simulink model "ctrl_student_HI_backup"  (R2015a)
settings: Solver=ode4  StartTime=0.0  StopTime=inf  FixedStep=0.01  RelTol=1e-3
undefined symbols (not defined in the file or in its folder): now, Par
(part 2 of 2)

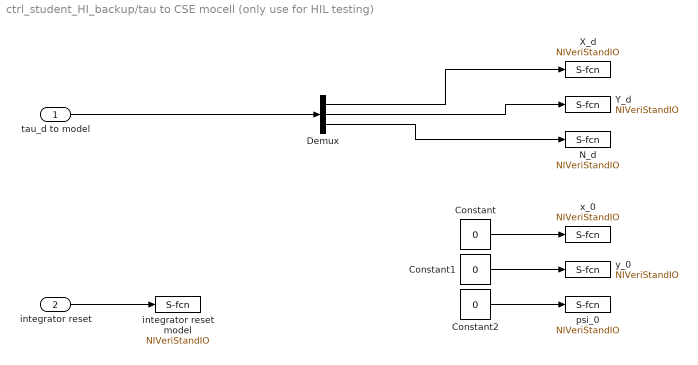
== system ctrl_student_HI_backup/tau to CSE mocell (only use for HIL testing) ==
  tau_d to model : Inport
  integrator reset : Inport  Port=2
  Constant : Constant  Value=0
  Constant1 : Constant  Value=0
  Constant2 : Constant  Value=0
  Demux : Demux  Outputs=3
  N_d : S-Function  Priority=2  FunctionName=NIVeriStandIO  Parameters=width dtype portnum stime stype btype  mask(NI VeriStand Outport){portnum=2, width=-1, stime=-1, dtype=auto, stype=auto, btype=0}
      mask prompts: portnum "Port number:"; width "Port dimensions (-1 for dynamically sized):"; stime "Sample time (-1 for inherited):"; dtype "Data type:"; stype "Signal type:"; btype "Block type:"
      mask help: Use this outport on any level of nested subsystems to allow NI VeriStand software to map signals to it.
      mask init:
      | NIVeriStandIO_init;
      settings: CopyFcn=NIVeriStand_MDL_functions('', 'IO_copy');  DeleteFcn=NIVeriStand_MDL_functions('', 'IO_delete');  MoveFcn=set_param(gcb, 'Mask', 'on');
      mask Callback portnum: NIVeriStand_MDL_functions('', 'IO_setportnum');
      mask TypeOptions dtype: auto | double | single | int8 | uint8 | int16 | uint16 | int32 | uint32 | boolean
      mask Callback dtype: NIVeriStand_MDL_functions('', 'IO_booleansignal');
      mask TypeOptions stype: auto | real | complex
      mask Display:
      | patch([-x x], [-y y], [.90980 .81960 .32156]);
      | plot([xrad -x x xrad], [yrad -y y yrad]);
      | fprintf('NI Out%d', portnum);
  X_d : S-Function  Priority=1  FunctionName=NIVeriStandIO  Parameters=width dtype portnum stime stype btype  mask(NI VeriStand Outport){portnum=1, width=-1, stime=-1, dtype=auto, stype=auto, btype=0}
      mask prompts: portnum "Port number:"; width "Port dimensions (-1 for dynamically sized):"; stime "Sample time (-1 for inherited):"; dtype "Data type:"; stype "Signal type:"; btype "Block type:"
      mask help: Use this outport on any level of nested subsystems to allow NI VeriStand software to map signals to it.
      mask init:
      | NIVeriStandIO_init;
      settings: CopyFcn=NIVeriStand_MDL_functions('', 'IO_copy');  DeleteFcn=NIVeriStand_MDL_functions('', 'IO_delete');  MoveFcn=set_param(gcb, 'Mask', 'on');
      mask Callback portnum: NIVeriStand_MDL_functions('', 'IO_setportnum');
      mask TypeOptions dtype: auto | double | single | int8 | uint8 | int16 | uint16 | int32 | uint32 | boolean
      mask Callback dtype: NIVeriStand_MDL_functions('', 'IO_booleansignal');
      mask TypeOptions stype: auto | real | complex
      mask Display:
      | patch([-x x], [-y y], [.90980 .81960 .32156]);
      | plot([xrad -x x xrad], [yrad -y y yrad]);
      | fprintf('NI Out%d', portnum);
  Y_d : S-Function  Priority=3  FunctionName=NIVeriStandIO  Parameters=width dtype portnum stime stype btype  mask(NI VeriStand Outport){portnum=3, width=-1, stime=-1, dtype=auto, stype=auto, btype=0}
      mask prompts: portnum "Port number:"; width "Port dimensions (-1 for dynamically sized):"; stime "Sample time (-1 for inherited):"; dtype "Data type:"; stype "Signal type:"; btype "Block type:"
      mask help: Use this outport on any level of nested subsystems to allow NI VeriStand software to map signals to it.
      mask init:
      | NIVeriStandIO_init;
      settings: CopyFcn=NIVeriStand_MDL_functions('', 'IO_copy');  DeleteFcn=NIVeriStand_MDL_functions('', 'IO_delete');  MoveFcn=set_param(gcb, 'Mask', 'on');
      mask Callback portnum: NIVeriStand_MDL_functions('', 'IO_setportnum');
      mask TypeOptions dtype: auto | double | single | int8 | uint8 | int16 | uint16 | int32 | uint32 | boolean
      mask Callback dtype: NIVeriStand_MDL_functions('', 'IO_booleansignal');
      mask TypeOptions stype: auto | real | complex
      mask Display:
      | patch([-x x], [-y y], [.90980 .81960 .32156]);
      | plot([xrad -x x xrad], [yrad -y y yrad]);
      | fprintf('NI Out%d', portnum);
  integrator reset model : S-Function  Priority=7  FunctionName=NIVeriStandIO  Parameters=width dtype portnum stime stype btype  mask(NI VeriStand Outport){portnum=7, width=-1, stime=-1, dtype=auto, stype=auto, btype=0}
      mask prompts: portnum "Port number:"; width "Port dimensions (-1 for dynamically sized):"; stime "Sample time (-1 for inherited):"; dtype "Data type:"; stype "Signal type:"; btype "Block type:"
      mask help: Use this outport on any level of nested subsystems to allow NI VeriStand software to map signals to it.
      mask init:
      | NIVeriStandIO_init;
      settings: CopyFcn=NIVeriStand_MDL_functions('', 'IO_copy');  DeleteFcn=NIVeriStand_MDL_functions('', 'IO_delete');  MoveFcn=set_param(gcb, 'Mask', 'on');
      mask Callback portnum: NIVeriStand_MDL_functions('', 'IO_setportnum');
      mask TypeOptions dtype: auto | double | single | int8 | uint8 | int16 | uint16 | int32 | uint32 | boolean
      mask Callback dtype: NIVeriStand_MDL_functions('', 'IO_booleansignal');
      mask TypeOptions stype: auto | real | complex
      mask Display:
      | patch([-x x], [-y y], [.90980 .81960 .32156]);
      | plot([xrad -x x xrad], [yrad -y y yrad]);
      | fprintf('NI Out%d', portnum);
  "psi_0 " : S-Function  Priority=4  FunctionName=NIVeriStandIO  Parameters=width dtype portnum stime stype btype  mask(NI VeriStand Outport){portnum=4, width=-1, stime=-1, dtype=auto, stype=auto, btype=0}
      mask prompts: portnum "Port number:"; width "Port dimensions (-1 for dynamically sized):"; stime "Sample time (-1 for inherited):"; dtype "Data type:"; stype "Signal type:"; btype "Block type:"
      mask help: Use this outport on any level of nested subsystems to allow NI VeriStand software to map signals to it.
      mask init:
      | NIVeriStandIO_init;
      settings: CopyFcn=NIVeriStand_MDL_functions('', 'IO_copy');  DeleteFcn=NIVeriStand_MDL_functions('', 'IO_delete');  MoveFcn=set_param(gcb, 'Mask', 'on');
      mask Callback portnum: NIVeriStand_MDL_functions('', 'IO_setportnum');
      mask TypeOptions dtype: auto | double | single | int8 | uint8 | int16 | uint16 | int32 | uint32 | boolean
      mask Callback dtype: NIVeriStand_MDL_functions('', 'IO_booleansignal');
      mask TypeOptions stype: auto | real | complex
      mask Display:
      | patch([-x x], [-y y], [.90980 .81960 .32156]);
      | plot([xrad -x x xrad], [yrad -y y yrad]);
      | fprintf('NI Out%d', portnum);
  x_0 : S-Function  Priority=5  FunctionName=NIVeriStandIO  Parameters=width dtype portnum stime stype btype  mask(NI VeriStand Outport){portnum=5, width=-1, stime=-1, dtype=auto, stype=auto, btype=0}
      mask prompts: portnum "Port number:"; width "Port dimensions (-1 for dynamically sized):"; stime "Sample time (-1 for inherited):"; dtype "Data type:"; stype "Signal type:"; btype "Block type:"
      mask help: Use this outport on any level of nested subsystems to allow NI VeriStand software to map signals to it.
      mask init:
      | NIVeriStandIO_init;
      settings: CopyFcn=NIVeriStand_MDL_functions('', 'IO_copy');  DeleteFcn=NIVeriStand_MDL_functions('', 'IO_delete');  MoveFcn=set_param(gcb, 'Mask', 'on');
      mask Callback portnum: NIVeriStand_MDL_functions('', 'IO_setportnum');
      mask TypeOptions dtype: auto | double | single | int8 | uint8 | int16 | uint16 | int32 | uint32 | boolean
      mask Callback dtype: NIVeriStand_MDL_functions('', 'IO_booleansignal');
      mask TypeOptions stype: auto | real | complex
      mask Display:
      | patch([-x x], [-y y], [.90980 .81960 .32156]);
      | plot([xrad -x x xrad], [yrad -y y yrad]);
      | fprintf('NI Out%d', portnum);
  y_0 : S-Function  Priority=6  FunctionName=NIVeriStandIO  Parameters=width dtype portnum stime stype btype  mask(NI VeriStand Outport){portnum=6, width=-1, stime=-1, dtype=auto, stype=auto, btype=0}
      mask prompts: portnum "Port number:"; width "Port dimensions (-1 for dynamically sized):"; stime "Sample time (-1 for inherited):"; dtype "Data type:"; stype "Signal type:"; btype "Block type:"
      mask help: Use this outport on any level of nested subsystems to allow NI VeriStand software to map signals to it.
      mask init:
      | NIVeriStandIO_init;
      settings: CopyFcn=NIVeriStand_MDL_functions('', 'IO_copy');  DeleteFcn=NIVeriStand_MDL_functions('', 'IO_delete');  MoveFcn=set_param(gcb, 'Mask', 'on');
      mask Callback portnum: NIVeriStand_MDL_functions('', 'IO_setportnum');
      mask TypeOptions dtype: auto | double | single | int8 | uint8 | int16 | uint16 | int32 | uint32 | boolean
      mask Callback dtype: NIVeriStand_MDL_functions('', 'IO_booleansignal');
      mask TypeOptions stype: auto | real | complex
      mask Display:
      | patch([-x x], [-y y], [.90980 .81960 .32156]);
      | plot([xrad -x x xrad], [yrad -y y yrad]);
      | fprintf('NI Out%d', portnum);
  wires:
  tau_d to model/1 -> Demux/1
  Demux/1 -> X_d/1
  Demux/2 -> Y_d/1
  Demux/3 -> N_d/1
  Constant2/1 -> "psi_0 "/1
  Constant1/1 -> y_0/1
  Constant/1 -> x_0/1
  integrator reset/1 -> integrator reset model/1

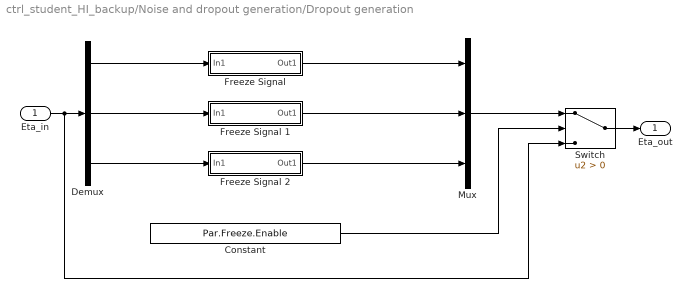
== system ctrl_student_HI_backup/Noise and dropout generation/Dropout generation ==
  Eta_in : Inport
  Constant : Constant  Value=Par.Freeze.Enable
  Demux : Demux  Outputs=3
  "Freeze Signal " : Subsystem
  Freeze Signal 1 : Subsystem
  Freeze Signal 2 : Subsystem
  Mux : Mux  Inputs=3
  Switch : Switch  Criteria=u2 > Threshold
  Eta_out : Outport
  wires:
  Eta_in/1 -> Switch/3, Demux/1
  Mux/1 -> Switch/1
  Demux/1 -> "Freeze Signal "/1(In1)
  "Freeze Signal "/1(Out1) -> Mux/1
  Freeze Signal 1/1(Out1) -> Mux/2
  Demux/2 -> Freeze Signal 1/1(In1)
  Demux/3 -> Freeze Signal 2/1(In1)
  Freeze Signal 2/1(Out1) -> Mux/3
  Constant/1 -> Switch/2
  Switch/1 -> Eta_out/1

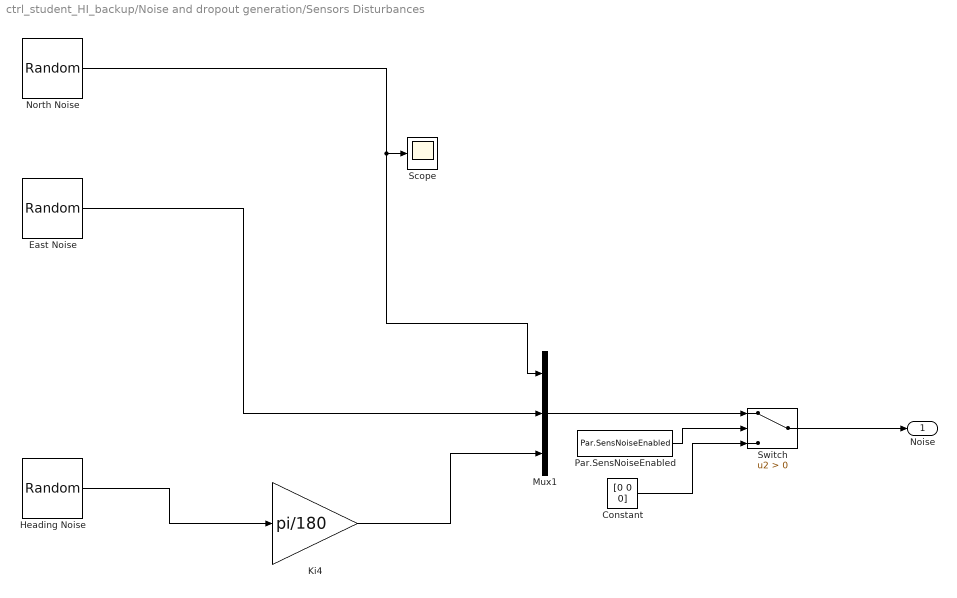
== system ctrl_student_HI_backup/Noise and dropout generation/Sensors Disturbances ==
  Constant : Constant  Value=[0 0 0]
  East Noise : RandomNumber  DisableCoverage=on  Variance=Par.Noise.Power  Seed=ceil(abs(5*round(abs(now*1e6 - fix(now*1e6))*1e5)))  SampleTime=Par.Sample_time  VectorParams1D=off
  Heading Noise : RandomNumber  DisableCoverage=on  Variance=Par.Noise.Power  Seed=ceil(abs(11*round(abs(now*1e6 - fix(now*1e6))*1e5)))  SampleTime=Par.Sample_time
  Ki4 : Gain  Gain=pi/180  RndMeth=Nearest
  Mux1 : Mux  Inputs=3
  North Noise : RandomNumber  DisableCoverage=on  Variance=Par.Noise.Power  Seed=ceil(abs(3*round(abs(now*1e6 - fix(now*1e6))*1e5)))  SampleTime=Par.Sample_time
  Par.SensNoiseEnabled : Constant  Value=Par.SensNoiseEnabled
  Scope : Scope
      settings: YMin=-0.51365  YMax=0.47143  SaveName=ScopeData2
  Switch : Switch  Criteria=u2 > Threshold
  Noise : Outport
  wires:
  East Noise/1 -> Mux1/2
  North Noise/1 -> Mux1/1, Scope/1
  Par.SensNoiseEnabled/1 -> Switch/2
  Switch/1 -> Noise/1
  Constant/1 -> Switch/3
  Mux1/1 -> Switch/1
  Heading Noise/1 -> Ki4/1
  Ki4/1 -> Mux1/3

== system ctrl_student_HI_backup/Signal Dropout detection/r ==
  detect droput : Inport
  nu : Inport  Port=2
  eta : Inport  Port=3
  Integrator : Integrator  ExternalReset=rising  InitialConditionSource=external
  Switch : Switch  Criteria=u2 ~= 0
  new_eta : Outport
  wires:
  Switch/1 -> new_eta/1
  nu/1 -> Integrator/1
  eta/1 -> Switch/3, Integrator/3
  detect droput/1 -> Switch/2, Integrator/2
  Integrator/1 -> Switch/1

== system ctrl_student_HI_backup/Signal Dropout detection/x ==
  detect droput : Inport
  nu : Inport  Port=2
  eta : Inport  Port=3
  Integrator : Integrator  ExternalReset=rising  InitialConditionSource=external
  Switch : Switch  Criteria=u2 ~= 0
  new_eta : Outport
  wires:
  Switch/1 -> new_eta/1
  nu/1 -> Integrator/1
  eta/1 -> Switch/3, Integrator/3
  detect droput/1 -> Switch/2, Integrator/2
  Integrator/1 -> Switch/1

== system ctrl_student_HI_backup/Signal Dropout detection/y ==
  detect droput : Inport
  nu : Inport  Port=2
  eta : Inport  Port=3
  Integrator : Integrator  ExternalReset=rising  InitialConditionSource=external
  Switch : Switch  Criteria=u2 ~= 0
  new_eta : Outport
  wires:
  Switch/1 -> new_eta/1
  nu/1 -> Integrator/1
  eta/1 -> Switch/3, Integrator/3
  detect droput/1 -> Switch/2, Integrator/2
  Integrator/1 -> Switch/1

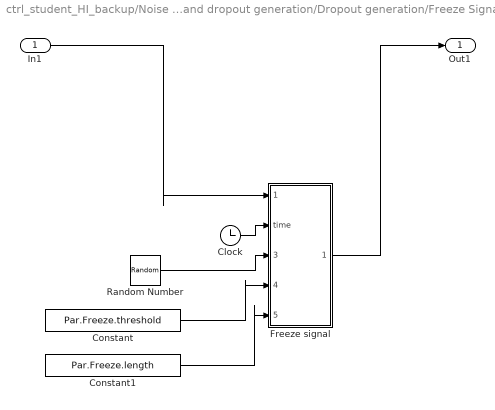
== system ctrl_student_HI_backup/Noise and dropout generation/Dropout generation/Freeze Signal  ==
  In1 : Inport
  Clock : Clock
  Constant : Constant  Value=Par.Freeze.threshold
  Constant1 : Constant  Value=Par.Freeze.length
  Freeze signal : MATLAB Function  TreatAsAtomicUnit=on
  Random Number : RandomNumber  Seed=ceil(abs(5*round(abs(now*1e6 - fix(now*1e6))*1e5)))  SampleTime=Par.Sample_time
  Out1 : Outport
  wires:
  Constant1/1 -> Freeze signal/5(length)
  In1/1 -> Freeze signal/1(eta_in)
  Freeze signal/1(eta_out) -> Out1/1
  Constant/1 -> Freeze signal/4(threshold)
  Clock/1 -> Freeze signal/2(time)
  Random Number/1 -> Freeze signal/3(random_value)

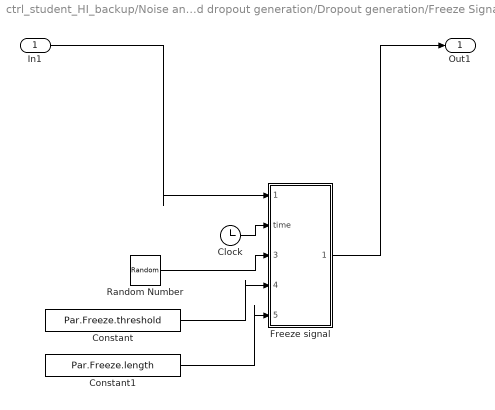
== system ctrl_student_HI_backup/Noise and dropout generation/Dropout generation/Freeze Signal 1 ==
  In1 : Inport
  Clock : Clock
  Constant : Constant  Value=Par.Freeze.threshold
  Constant1 : Constant  Value=Par.Freeze.length
  Freeze signal : MATLAB Function  TreatAsAtomicUnit=on
  Random Number : RandomNumber  Seed=ceil(abs(5*round(abs(now*1e6 - fix(now*1e6))*1e5)))  SampleTime=Par.Sample_time
  Out1 : Outport
  wires:
  Constant1/1 -> Freeze signal/5(length)
  In1/1 -> Freeze signal/1(eta_in)
  Freeze signal/1(eta_out) -> Out1/1
  Constant/1 -> Freeze signal/4(threshold)
  Clock/1 -> Freeze signal/2(time)
  Random Number/1 -> Freeze signal/3(random_value)

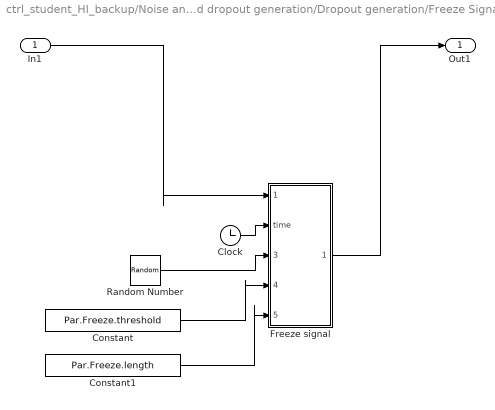
== system ctrl_student_HI_backup/Noise and dropout generation/Dropout generation/Freeze Signal 2 ==
  In1 : Inport
  Clock : Clock
  Constant : Constant  Value=Par.Freeze.threshold
  Constant1 : Constant  Value=Par.Freeze.length
  Freeze signal : MATLAB Function  TreatAsAtomicUnit=on
  Random Number : RandomNumber  Seed=ceil(abs(5*round(abs(now*1e6 - fix(now*1e6))*1e5)))  SampleTime=Par.Sample_time
  Out1 : Outport
  wires:
  Constant1/1 -> Freeze signal/5(length)
  In1/1 -> Freeze signal/1(eta_in)
  Freeze signal/1(eta_out) -> Out1/1
  Constant/1 -> Freeze signal/4(threshold)
  Clock/1 -> Freeze signal/2(time)
  Random Number/1 -> Freeze signal/3(random_value)

== matlab function ctrl_student_HI_backup/Thrust Allocation/MATLAB Function ==
  data: X input; u output; Y input; N input; invT input
function u = fcn(X, Y, N, invT)
%#codegen
u = [0 0 0]';
u = invT*[X, Y, N]';

== matlab function ctrl_student_HI_backup/Surge Observer/inside of integral ==
  data: psi input; k_psi input; X input; u_hat input; integral output
function integral = fcn(psi, k_psi, X, u_hat)
%#codegen
X_u = -.6555;
X_uu = .3545;
X_uuu = -3.787;
m_11 = 16.79;
d_11 = -X_u -X_uu*abs(u_hat) - X_uuu*u_hat^2;
integral = -d_11*u_hat/m_11 + X/m_11 - k_psi*(cos(psi) + sin(psi))*u_hat;
end

== matlab function ctrl_student_HI_backup/Workspace saturation/MATLAB Function ==
  data: eta input; tau_out output; tau_in input; x_min input; x_max input; y_min input; y_max input; threshold input; scale input
function tau_out = fcn(eta, tau_in, x_min, x_max, y_min, y_max, threshold, scale)
%#codegen
R = [cos(eta(3)) sin(eta(3)) 0 ; -sin(eta(3)) cos(eta(3)) 0; 0 0 1];

tau_NED = R*tau_in;
tau_NED_out = tau_NED;

%check if x is above limits
if (eta(1) > x_max)
    %x is above of the limit
    epsilon = scale*(eta(1) - x_max)/threshold;
    tau_NED_out(1) = -epsilon + tau_NED(1)*(1-epsilon);
end
%check if x is below limits
if (eta(1) < x_min)
    %x is below of the limit
    epsilon = scale*(eta(1) - x_min)/threshold;
    tau_NED_out(1) = -epsilon + tau_NED(1)*(1+epsilon);
end
%check if y is above limits
if (eta(2) > y_max)
    %x is above of the limit
    epsilon = scale*(eta(2) - y_max)/threshold;
    tau_NED_out(2) = -epsilon + tau_NED(2)*(1-epsilon);
end
%check if y is above limits
if (eta(2) < y_min)
    %x is above of the limit
    epsilon = scale*(eta(2) - y_min)/threshold;
    tau_NED_out(2) = -epsilon + tau_NED(2)*(1+epsilon);
end
tau_out = R'*tau_NED_out;
end

== matlab function ctrl_student_HI_backup/Sixaxis2force/MATLAB Function1 ==
  data: u input; u_VSP output; alpha_VSP output; u_BT output
function [u_VSP, alpha_VSP, u_BT]    = fcn(u)
u_VSP = min([sqrt(u(1)^2 + u(2)^2), 1]);
alpha_VSP = atan2(u(2), u(1));
u_BT = u(3);

== matlab function ctrl_student_HI_backup/Surge Observer/k_psi ==
  data: psi input; k_psi input; K_psi output
function K_psi = fcn(psi,k_psi)
%#codegen
K_psi = k_psi*sign(sin(psi) + cos(psi));
% y = u;

== matlab function ctrl_student_HI_backup/Signal Dropout detection/Detect droput ==
  data: dropout_log output; eta_in input; dropout output
function [dropout_log, dropout]  = fcn(eta_in)
persistent eta_old;
if isempty(eta_old)
    eta_old = eta_in;
end
dropout_log = zeros(3, 1);
dropout = (eta_in - eta_old) == 0;
for i = 1:3
    if dropout(i)
        dropout_log(i) = 1.00;
    end
end
eta_old = eta_in;
end

== matlab function ctrl_student_HI_backup/Noise and dropout generation/Dropout generation/Freeze Signal /Freeze signal ==
  data: eta_in input; eta_out output; time input; random_value input; threshold input; length input
function eta_out = fcn(eta_in, time, random_value, threshold, length)
persistent eta t_1;
if isempty(eta)
    eta = eta_in;
    t_1 = 0;
end

if random_value > threshold
    t_1 = time + length*(0.5*rand+0.5);
end
if time>=t_1
    eta = eta_in;
end

eta_out = eta;
end

== matlab function ctrl_student_HI_backup/Noise and dropout generation/Dropout generation/Freeze Signal 1/Freeze signal ==
  data: eta_in input; eta_out output; time input; random_value input; threshold input; length input
function eta_out = fcn(eta_in, time, random_value, threshold, length)
persistent eta t_1;
if isempty(eta)
    eta = eta_in;
    t_1 = 0;
end

if random_value > threshold
    t_1 = time + length*(0.5*rand+0.5);
end
if time>=t_1
    eta = eta_in;
end

eta_out = eta;
end

== matlab function ctrl_student_HI_backup/Noise and dropout generation/Dropout generation/Freeze Signal 2/Freeze signal ==
  data: eta_in input; eta_out output; time input; random_value input; threshold input; length input
function eta_out = fcn(eta_in, time, random_value, threshold, length)
persistent eta t_1;
if isempty(eta)
    eta = eta_in;
    t_1 = 0;
end

if random_value > threshold
    t_1 = time + length*(0.5*rand+0.5);
end
if time>=t_1
    eta = eta_in;
end

eta_out = eta;
end
